simulink library "uORBlib"  (R2021a)
settings: Solver=VariableStepAuto  StartTime=0.0  StopTime=10.0  RelTol=1e-3
undefined symbols (not defined in the file or in its folder): nuttx
settings Model: Creator=asanchez  LastModifiedBy=asanchez

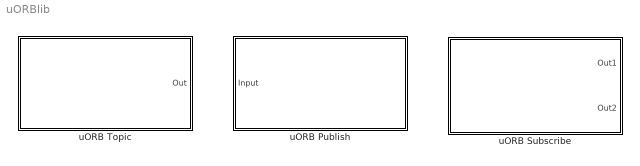
== system uORBlib ==
  uORB Publish : Subsystem  mask(Nuttx uORB Publish){uORBTopic=log_message, selectInstance=log_message}
      mask prompts: uORBTopic "Topic :"
      mask init:
      | nuttx.internal.block.PublishBlockMask.dispatch('maskInitialize',gcb);
      mask Callback uORBTopic: nuttx.internal.block.PublishBlockMask.dispatch('topicEdit',gcb);
      mask TypeOptions selectInstance: log_message
      mask DialogControl Container4 Prompt: Main
      mask DialogControl topicSelecBtn Prompt: Select
      mask DialogControl topicSelecBtn Callback: nuttx.internal.block.PublishBlockMask.dispatch('topicSelect',gcb);
      mask DialogControl Container5 Prompt: Advanced
      mask Display:
      | color('blue');
      | text(0.2, 0.90, 'Nuttx', 'horizontalAlignment', 'right');
      | color('black');
      | text(0.5, 0.60, 'uORB Publish', 'horizontalAlignment', 'center');
      | if length(uORBTopic) > 20
      |   text(0.95, 0.15, uORBTopic, 'horizontalAlignment', 'right');
      | else
      |   text(0.5, 0.15, uORBTopic, 'horizontalAlignment', 'center');
      | end
      | port_label('input', 1, 'Msg');
  uORB Subscribe : Subsystem  mask(Nuttx uORB Read){uORBTopic=log_message, selectInstance=log_message, SampleTime=0.001, BlockingMode=off, BlockTimeout=1e-3}
      mask prompts: uORBTopic "nuttx:blockmask:TopicPrompt"; selectInstance "nuttx:blockmask:SelectInstance"; SampleTime "nuttx:blockmask:SampleTimePrompt"; BlockingMode "Wait until data received"; BlockTimeout "Timeout in seconds:"
      mask init:
      | nuttx.internal.block.SubscribeBlockMask.dispatch('maskInitialize', gcb);
      mask Callback uORBTopic: nuttx.internal.block.SubscribeBlockMask.dispatch('topicEdit', gcb);
      mask TypeOptions selectInstance: log_message
      mask TypeOptions SampleTime: SourceBlock/SampleTime
      mask TypeOptions BlockingMode: SourceBlock/BlockingMode
      mask Callback BlockingMode: nuttx.internal.block.SubscribeBlockMask.dispatch('blockingModeSelect', gcb);
      mask TypeOptions BlockTimeout: SourceBlock/BlockTimeout
      mask DialogControl ContainerMain Prompt: Main
      mask DialogControl topicSelectButton Prompt: Select
      mask DialogControl topicSelectButton Callback: nuttx.internal.block.SubscribeBlockMask.dispatch('topicSelect', gcb);
      mask DialogControl ContainerAdvanced Prompt: Advanced
      mask Display:
      | color('blue');
      | text(0.2, 0.90, 'Nuttx', 'horizontalAlignment', 'right');
      | color('black');
      | text(0.5, 0.60, 'uORB Subscribe', 'horizontalAlignment', 'center');
      | if length(uORBTopic) > 16
      |   text(0.83, 0.15, uORBTopic, 'horizontalAlignment', 'right');
      | else
      |   text(0.5, 0.15, uORBTopic, 'horizontalAlignment', 'center');
      | end
      | port_label('output', 1, 'Status');
      | port_label('output', 2, 'Msg');
  uORB Topic : Subsystem  SystemSampleTime=SampleTime  mask(uORB Message){uORBTopic=log_message, SampleTime=inf, selectInstance=log_message}
      mask prompts: uORBTopic "Topic :"; SampleTime "Simulink:blkprm_prompts:AllBlksSampleTime"
      mask init:
      | nuttx.internal.block.MessageBlockMask.dispatch('maskInitialize', gcb);
      mask Callback uORBTopic: nuttx.internal.block.MessageBlockMask.dispatch('topicEdit', gcb);
      mask TypeOptions SampleTime: SystemSampleTime
      mask TypeOptions selectInstance: log_message
      mask DialogControl Container5 Prompt: Main
      mask DialogControl topicSelectBtn Prompt: Select
      mask DialogControl topicSelectBtn Callback: nuttx.internal.block.MessageBlockMask.dispatch('topicSelect', gcb);
      mask DialogControl SampleTime Prompt: Sample time (-1 for inherited):
      mask Display:
      | color('blue');
      | text(0.2, 0.90, 'Nuttx', 'horizontalAlignment', 'right');
      | color('black');
      | text(0.5, 0.60, 'uORB Message', 'horizontalAlignment', 'center');
      | 
      | if length(uORBTopic) > 16
      |   text(0.83, 0.15, uORBTopic, 'horizontalAlignment', 'right');
      | else
      |   text(0.5, 0.15, uORBTopic, 'horizontalAlignment', 'center');
      | end
      | 
      | port_label('output', 1, 'Msg');

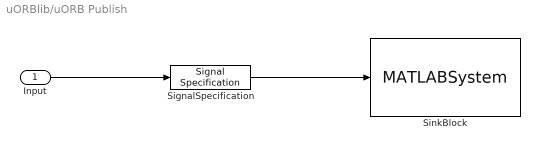
== system uORBlib/uORB Publish ==
  Input : Inport
  SignalSpecification : SignalSpecification  OutDataTypeStr=Bus: nuttx_Bus_log_message  BusOutputAsStruct=on
      settings: LockScale=on
  SinkBlock : MATLABSystem  System=nuttx.internal.block.Publisher  uORBTopic=log_message  MessageQueueLen=1  uORBTopicInstance=log_message  SLBusName=nuttx_Bus_log_message
      mask Type: nuttx.internal.block.Publisher
      mask Display: disp('Publisher');
  wires:
  Input/1 -> SignalSpecification/1
  SignalSpecification/1 -> SinkBlock/1

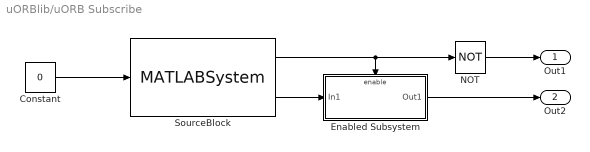
== system uORBlib/uORB Subscribe ==
  Constant : Constant  Value=0  OutDataTypeStr=Bus: nuttx_Bus_log_message
  Enabled Subsystem : Subsystem  TreatAsAtomicUnit=on
  NOT : Logic  Operator=NOT  IconShape=distinctive  AllPortsSameDT=off  OutDataTypeStr=boolean
  SourceBlock : MATLABSystem  InitFcn=nuttx.internal.block.SubscribeBlockMask.dispatch('sysobjInitFcn', gcb);  System=nuttx.internal.block.Subscriber  uORBTopic=log_message  uORBTopicInstance=log_message  SLBusName=nuttx_Bus_log_message  SampleTime=SampleTime  BlockingMode=off  BlockTimeout=BlockTimeout
      mask Type: nuttx.internal.block.Subscriber
      mask Display:
      | disp('Subscriber');
      | port_label('input',1,'busstruct');
      | port_label('output',1,'isNewData');
      | port_label('output',2,'msg');
  Out1 : Outport  SampleTime=0.001
  Out2 : Outport  Port=2
  wires:
  Constant/1 -> SourceBlock/1
  SourceBlock/2 -> Enabled Subsystem/1(In1)
  SourceBlock/1 -> NOT/1, Enabled Subsystem/Enable
  NOT/1 -> Out1/1
  Enabled Subsystem/1(Out1) -> Out2/1

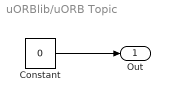
== system uORBlib/uORB Topic ==
  Constant : Constant  InitFcn=nuttx.internal.block.MessageBlockMask.dispatch('constantBlkInitFcn', gcb);  Value=0  OutDataTypeStr=Bus: nuttx_Bus_log_message  SampleTime=SampleTime
  Out : Outport  VectorParamsAs1DForOutWhenUnconnected=off
  wires:
  Constant/1 -> Out/1

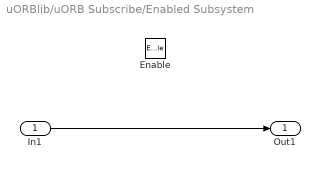
== system uORBlib/uORB Subscribe/Enabled Subsystem ==
  In1 : Inport
  Enable : EnablePort
  Out1 : Outport
  wires:
  In1/1 -> Out1/1
